simulink model "AirCtl_Gov"  (R2016b)
settings: configuration reference "CodeGenConfigSet" (kept outside this file)
values from neighbouring files (symbols this model uses):
  AirCtl_facParAirTemp_CUR = Calibration.Parameter    [init_AirCtl_Gov.m]    (also in init_AirCtl_Gov_SIL.m = Simulink.Parameter)
  AirCtl_facParAirTemp_CURX = Calibration.Parameter    [init_AirCtl_Gov.m]    (also in init_AirCtl_Gov_SIL.m = Simulink.Parameter)
  AirCtl_facParBas_MAP = Calibration.Parameter    [init_AirCtl_Gov.m]    (also in init_AirCtl_Gov_SIL.m = Simulink.Parameter)
  AirCtl_facParBas_MAPX = Calibration.Parameter    [init_AirCtl_Gov.m]    (also in init_AirCtl_Gov_SIL.m = Simulink.Parameter)
  AirCtl_facParBas_MAPY = Calibration.Parameter    [init_AirCtl_Gov.m]    (also in init_AirCtl_Gov_SIL.m = Simulink.Parameter)
  AirCtl_KdNrm_C = Calibration.Parameter    [init_AirCtl_Gov.m]    (also in init_AirCtl_Gov_SIL.m = Simulink.Parameter)
  AirCtl_KIconv_C = Calibration.Parameter    [init_AirCtl_Gov.m]    (also in init_AirCtl_Gov_SIL.m = Simulink.Parameter)
  AirCtl_KiNegNrm_C = Calibration.Parameter    [init_AirCtl_Gov.m]    (also in init_AirCtl_Gov_SIL.m = Simulink.Parameter)
  AirCtl_KiNrm_C = Calibration.Parameter    [init_AirCtl_Gov.m]    (also in init_AirCtl_Gov_SIL.m = Simulink.Parameter)
  AirCtl_KiPosNrm_C = Calibration.Parameter    [init_AirCtl_Gov.m]    (also in init_AirCtl_Gov_SIL.m = Simulink.Parameter)
  AirCtl_KiWinNegNrm_C = Calibration.Parameter    [init_AirCtl_Gov.m]    (also in init_AirCtl_Gov_SIL.m = Simulink.Parameter)
  AirCtl_KiWinPosNrm_C = Calibration.Parameter    [init_AirCtl_Gov.m]    (also in init_AirCtl_Gov_SIL.m = Simulink.Parameter)
  AirCtl_KpNegNrm_C = Calibration.Parameter    [init_AirCtl_Gov.m]    (also in init_AirCtl_Gov_SIL.m = Simulink.Parameter)
  AirCtl_KpNrm_C = Calibration.Parameter    [init_AirCtl_Gov.m]    (also in init_AirCtl_Gov_SIL.m = Simulink.Parameter)
  AirCtl_KpPosNrm_C = Calibration.Parameter    [init_AirCtl_Gov.m]    (also in init_AirCtl_Gov_SIL.m = Simulink.Parameter)
  AirCtl_KpWinNegNrm_C = Calibration.Parameter    [init_AirCtl_Gov.m]    (also in init_AirCtl_Gov_SIL.m = Simulink.Parameter)
  AirCtl_KpWinPosNrm_C = Calibration.Parameter    [init_AirCtl_Gov.m]    (also in init_AirCtl_Gov_SIL.m = Simulink.Parameter)
  AirCtl_numAirTempGov_C = Calibration.Parameter    [init_AirCtl_Gov.m]    (also in init_AirCtl_Gov_SIL.m = Simulink.Parameter)
  AirCtl_rEGR_MAP = Calibration.Parameter    [init_AirCtl_Gov.m]    (also in init_AirCtl_Gov_SIL.m = Simulink.Parameter)
  AirCtl_rEGR_MAPX = Calibration.Parameter    [init_AirCtl_Gov.m]    (also in init_AirCtl_Gov_SIL.m = Simulink.Parameter)
  AirCtl_rEGR_MAPY = Calibration.Parameter    [init_AirCtl_Gov.m]    (also in init_AirCtl_Gov_SIL.m = Simulink.Parameter)
  AirCtl_rGovMax_C = Calibration.Parameter    [init_AirCtl_Gov.m]    (also in init_AirCtl_Gov_SIL.m = Simulink.Parameter)
  AirCtl_rGovMin_C = Calibration.Parameter    [init_AirCtl_Gov.m]    (also in init_AirCtl_Gov_SIL.m = Simulink.Parameter)
  AirCtl_rIGovLimHi_C = Calibration.Parameter    [init_AirCtl_Gov.m]    (also in init_AirCtl_Gov_SIL.m = Simulink.Parameter)
  AirCtl_rIGovLimLo_C = Calibration.Parameter    [init_AirCtl_Gov.m]    (also in init_AirCtl_Gov_SIL.m = Simulink.Parameter)
  AirCtl_rTransCor_MAP = Calibration.Parameter    [init_AirCtl_Gov.m]    (also in init_AirCtl_Gov_SIL.m = Simulink.Parameter)
  AirCtl_rTransCor_MAPX = Calibration.Parameter    [init_AirCtl_Gov.m]    (also in init_AirCtl_Gov_SIL.m = Simulink.Parameter)
  AirCtl_rTransCor_MAPY = Calibration.Parameter    [init_AirCtl_Gov.m]    (also in init_AirCtl_Gov_SIL.m = Simulink.Parameter)
  AirCtl_rTVA_MAP = Calibration.Parameter    [init_AirCtl_Gov.m]    (also in init_AirCtl_Gov_SIL.m = Simulink.Parameter)
  AirCtl_rTVA_MAPX = Calibration.Parameter    [init_AirCtl_Gov.m]    (also in init_AirCtl_Gov_SIL.m = Simulink.Parameter)
  AirCtl_rTVA_MAPY = Calibration.Parameter    [init_AirCtl_Gov.m]    (also in init_AirCtl_Gov_SIL.m = Simulink.Parameter)
  AirCtl_stGov_C = Calibration.Parameter    [init_AirCtl_Gov.m]    (also in init_AirCtl_Gov_SIL.m = Simulink.Parameter)
  AirCtl_T1Nrm_C = Calibration.Parameter    [init_AirCtl_Gov.m]    (also in init_AirCtl_Gov_SIL.m = Simulink.Parameter)
undefined symbols (not defined in the file or in its folder): AirCtl_Gov_DT
libraries: CXLib x4
settings Model: Creator=Wollf  LastModifiedBy=zhulinfeng
settings ConfigSetRef: SourceLocation=Base Workspace

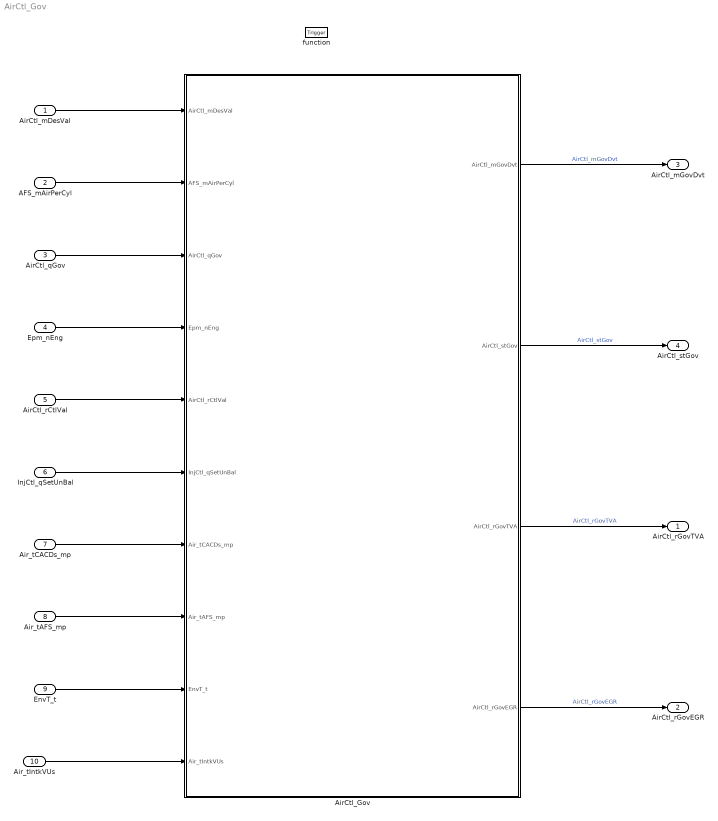
== system AirCtl_Gov ==
  AirCtl_mDesVal : Inport  Tag=mg/hub  Description=Desired air mass  OutMin=-15000  OutMax=15000  OutDataTypeStr=AirMass_mg_hub
  AFS_mAirPerCyl : Inport  Tag=mg/hub  Description=Air mass per cylinder  Port=2  OutMin=0  OutMax=16383  OutDataTypeStr=AirMass_mg_hub
  AirCtl_qGov : Inport  Tag=mg/hub  Description=Inner quantity for open-loop control of the exhaustgas recirculation control  Port=3  OutMin=-319  OutMax=319  OutDataTypeStr=FuelMass_mg_hub
  Epm_nEng : Inport  Tag=rpm  Description=Engine speed  Port=4  OutMin=0  OutMax=6000  OutDataTypeStr=EngSpeed_rpm
  AirCtl_rCtlVal : Inport  Tag=%  Description=Stationary part of controlled variable  Port=5  OutMin=-100  OutMax=100  OutDataTypeStr=Prc_100_rate
  InjCtl_qSetUnBal : Inport  Tag=mg/hub  Description=Current injection quantity  Port=6  OutMin=-319  OutMax=319  OutDataTypeStr=FuelMass_mg_hub
  Air_tCACDs_mp : Inport  Tag=deg  Description=Charge-air temperature downstream from charge-air cooler  Port=7  OutMin=-200  OutMax=200  OutDataTypeStr=Temp_deg
  Air_tAFS_mp : Inport  Tag=deg  Description=Induction air temperature at the HFM  Port=8  OutMin=-200  OutMax=200  OutDataTypeStr=Temp_deg
  EnvT_t : Inport  Tag=deg  Description=Environmental temperature  Port=9  OutMin=-200  OutMax=200  OutDataTypeStr=Temp_deg
  Air_tIntkVUs : Inport  Tag=deg  Description=Intake air temperature upstream of the inlet valve  Port=10  OutMin=-200  OutMax=200  OutDataTypeStr=Temp_deg
  function : TriggerPort  TriggerType=function-call  VariantControl=Variant
  AirCtl_Gov : Subsystem
  AirCtl_rGovTVA : Outport  Tag=%  Description=Opening for intake throttle (TVA)  OutMin=-100  OutMax=100  OutDataTypeStr=Prc_100_rate
  AirCtl_rGovEGR : Outport  Tag=%  Description=Setpoint position of the exhaust-gas recirculation valve from the exhaust-gas recirculation control  Port=2  OutMin=-100  OutMax=100  OutDataTypeStr=Prc_100_rate
  AirCtl_mGovDvt : Outport  Tag=mg/hub  Description=Deviation of Air mass  Port=3  OutMin=-15000  OutMax=15000  OutDataTypeStr=AirMass_mg_hub
  AirCtl_stGov : Outport  Description=Status of the exhaust-gas recirculation control  Port=4  OutMin=0  OutMax=255  OutDataTypeStr=State_uint8
  wires:
  AirCtl_mDesVal/1 -> AirCtl_Gov/1(AirCtl_mDesVal)
  AFS_mAirPerCyl/1 -> AirCtl_Gov/2(AFS_mAirPerCyl)
  AirCtl_qGov/1 -> AirCtl_Gov/3(AirCtl_qGov)
  Epm_nEng/1 -> AirCtl_Gov/4(Epm_nEng)
  AirCtl_rCtlVal/1 -> AirCtl_Gov/5(AirCtl_rCtlVal)
  InjCtl_qSetUnBal/1 -> AirCtl_Gov/6(InjCtl_qSetUnBal)
  Air_tCACDs_mp/1 -> AirCtl_Gov/7(Air_tCACDs_mp)
  Air_tAFS_mp/1 -> AirCtl_Gov/8(Air_tAFS_mp)
  EnvT_t/1 -> AirCtl_Gov/9(EnvT_t)
  Air_tIntkVUs/1 -> AirCtl_Gov/10(Air_tIntkVUs)
  AirCtl_Gov/1(AirCtl_mGovDvt) -> AirCtl_mGovDvt/1  "AirCtl_mGovDvt"
  AirCtl_Gov/2(AirCtl_stGov) -> AirCtl_stGov/1  "AirCtl_stGov"
  AirCtl_Gov/3(AirCtl_rGovTVA) -> AirCtl_rGovTVA/1  "AirCtl_rGovTVA"
  AirCtl_Gov/4(AirCtl_rGovEGR) -> AirCtl_rGovEGR/1  "AirCtl_rGovEGR"

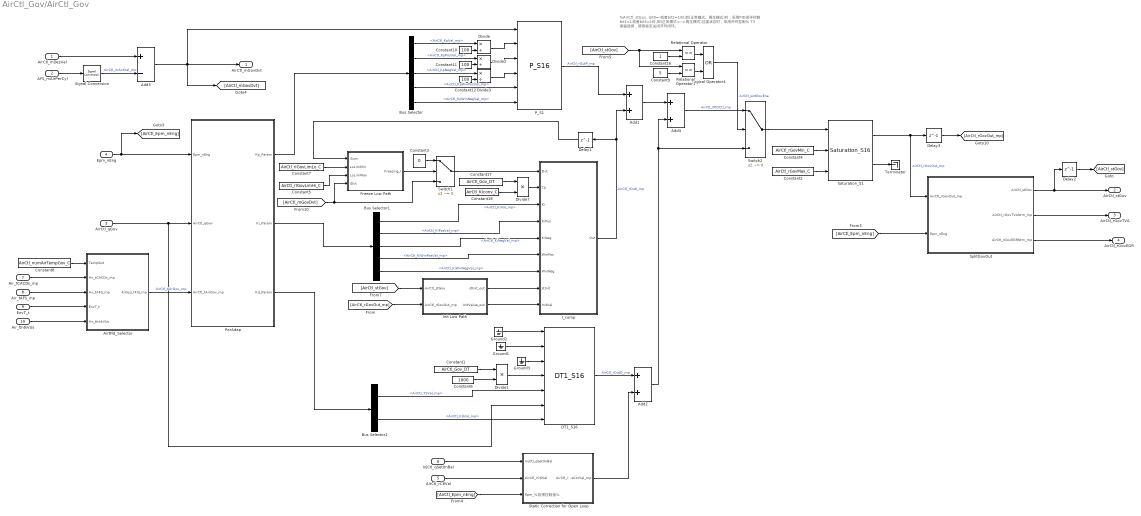
== system AirCtl_Gov/AirCtl_Gov ==
  note: %AirCtl_stGov,
      | bit0=1或者bit2=1时,即(正常模式、再生模式)时，采用PID闭环控制
      | bit1=1或者bit3=1时,即(正常模式<-->再生模式)过渡状态时，采用开环控制%
      | T3 保留选择，使用标定关闭开环闭环。
  note: %前馈控制值%
  AirCtl_mDesVal : Inport  Tag=mg/hub  Description=Desired air mass  OutDataTypeStr=AirMass_mg_hub
  AFS_mAirPerCyl : Inport  Tag=mg/hub  Description=Air mass per cylinder  Port=2
  AirCtl_qGov : Inport  Tag=mg/hub  Description=Inner quantity for open-loop control of the exhaustgas recirculation control  Port=3
  Epm_nEng : Inport  Tag=rpm  Description=Engine speed  Port=4
  AirCtl_rCtlVal : Inport  Tag=%  Description=Stationary part of controlled variable  Port=5
  InjCtl_qSetUnBal : Inport  Tag=mg/hub  Description=Current injection quantity  Port=6
  Air_tCACDs_mp : Inport  Tag=deg  Description=Charge-air temperature downstream from charge-air cooler  Port=7
  Air_tAFS_mp : Inport  Tag=deg  Description=Induction air temperature at the HFM  Port=8
  EnvT_t : Inport  Tag=deg  Description=Environmental temperature  Port=9
  Air_tIntkVUs : Inport  Tag=deg  Description=Intake air temperature upstream of the inlet valve  Port=10
  Add1 : Sum  SaturateOnIntegerOverflow=on  InputSameDT=on
  Add2 : Sum  SaturateOnIntegerOverflow=on  InputSameDT=on
  Add3 : Sum  Inputs=+-  SaturateOnIntegerOverflow=on  InputSameDT=on
  Add4 : Sum  SaturateOnIntegerOverflow=on  InputSameDT=on
  AirtFld_Selector : Subsystem
  Bus Selector : BusSelector  OutputSignals=AirCtl_KpVal_mp,AirCtl_KpPosVal_mp,AirCtl_KpNegVal_mp,AirCtl_KpWinPosVal_mp,AirCtl_KpWinNegVal_mp
  Bus Selector1 : BusSelector  OutputSignals=AirCtl_KiVal_mp,AirCtl_KiPosVal_mp,AirCtl_KiNegVal_mp,AirCtl_KiWinPosVal_mp,AirCtl_KiWinNegVal_mp
  Bus Selector2 : BusSelector  OutputSignals=AirCtl_T1Val_mp,AirCtl_KdVal_mp
  Constant1 : Constant  Value=AirCtl_Gov_DT
  Constant10 : Constant  Value=100  OutDataTypeStr=uint8
  Constant11 : Constant  Value=100  OutDataTypeStr=uint8
  Constant12 : Constant  Value=100  OutDataTypeStr=uint8
  Constant16 : Constant  OutDataTypeStr=Inherit: Inherit via back propagation
  Constant17 : Constant  Value=AirCtl_Gov_DT
  Constant18 : Constant  Value=AirCtl_KIconv_C
  Constant2 : Constant  Value=AirCtl_rGovMax_C
  Constant3 : Constant  Value=0  OutDataTypeStr=Inherit: Inherit via back propagation
  Constant4 : Constant  Value=AirCtl_rGovMin_C
  Constant5 : Constant  Value=AirCtl_rIGovLimHi_C
  Constant6 : Constant  Value=1000  OutDataTypeStr=uint32
  Constant7 : Constant  Value=AirCtl_rIGovLimLo_C
  Constant8 : Constant  Value=AirCtl_numAirTempGov_C
  Constant9 : Constant  Value=5  OutDataTypeStr=Inherit: Inherit via back propagation
  DT1_S16 : CXLib/DT1_S16
  Delay1 : Delay  DelayLength=1  InitialCondition=0
  Delay2 : Delay  DelayLength=1  InitialCondition=0
  Delay3 : Delay  DelayLength=1  InitialCondition=0
  Divide : Product  Inputs=*/  OutDataTypeStr=fixdt(1,32,2^-14,0)  SaturateOnIntegerOverflow=on
  Divide1 : Product  Inputs=**  OutDataTypeStr=Inherit: Inherit via back propagation  SaturateOnIntegerOverflow=on
  Divide2 : Product  Inputs=*/  OutDataTypeStr=fixdt(1,32,2^-14,0)  SaturateOnIntegerOverflow=on
  Divide3 : Product  Inputs=*/  OutDataTypeStr=fixdt(1,32,2^-14,0)  SaturateOnIntegerOverflow=on
  Divide7 : Product  Inputs=**  SaturateOnIntegerOverflow=on  OutDataTypeStr=Inherit: Same as first input
  Freeze Low Path : Subsystem
  Ground1 : Ground
  Ground2 : Ground
  Ground3 : Ground
  I_comp : Subsystem
  Init Low Path : Subsystem
  Logical Operator4 : Logic  Operator=OR  OutDataTypeStr=boolean
  P_S1 : CXLib/P_S16
  ParAdap : Subsystem
  Relational Operator : RelationalOperator  Operator===  OutDataTypeStr=boolean  RndMeth=Simplest
  Relational Operator1 : RelationalOperator  Operator===  OutDataTypeStr=boolean  RndMeth=Simplest
  Saturation_S1 : CXLib/Saturation_S16
  Signal Conversion : SignalConversion  OverrideOpt=off
  SplitGovOut : Subsystem
  Static Correction for Open Loop : Subsystem
  Switch1 : Switch  Criteria=u2 ~= 0  SaturateOnIntegerOverflow=on  InputSameDT=on
  Switch2 : Switch  Criteria=u2 ~= 0  SaturateOnIntegerOverflow=on  InputSameDT=on
  Terminator : Terminator
  AirCtl_mGovDvt : Outport  Tag=mg/hub  Description=Deviation of Air mass
  AirCtl_stGov : Outport  Description=Status of the exhaust-gas recirculation control  Port=2
  AirCtl_rGovTVA : Outport  Tag=%  Description=Opening for intake throttle (TVA)  Port=3
  AirCtl_rGovEGR : Outport  Tag=%  Description=Setpoint position of the exhaust-gas recirculation valve from the exhaust-gas recirculation control  Port=4
  wires:
  I_comp/1(Out) -> Add1/2, Delay1/1  "AirCtl_rOutI_mp"
  Bus Selector/1 -> Divide/1  "<AirCtl_KpVal_mp>"
  Static Correction for Open Loop/1(AirCtl_rTransCorVal_mp) -> Add2/2
  Bus Selector2/2 -> DT1_S16/7  "<AirCtl_KdVal_mp>"
  ParAdap/2(Ki_Param) -> Bus Selector1/1
  AirCtl_mDesVal/1 -> Add3/1
  ParAdap/1(Kp_Param) -> Bus Selector/1
  Delay1/1 -> Freeze Low Path/1(iSum)
  Constant6/1 -> Divide1/2
  Constant1/1 -> Divide1/1
  Delay3/1 -> [AirCtl_rGovOut_mp]
  Logical Operator4/1 -> Switch2/2  "AirCtl_swtGovEna"
  Constant5/1 -> Freeze Low Path/3(LoLimMax)
  [AirCtl_rGovOut_mp] -> Init Low Path/2(AirCtl_rGovOut_mp)
  [AirCtl_stGov] -> Init Low Path/1(AirCtl_stGov)
  [AirCtl_stGov] -> Relational Operator1/1, Relational Operator/1
  Constant7/1 -> Freeze Low Path/2(LoLimMin)
  Init Low Path/1(stInit_out) -> I_comp/8(stInit)
  Switch1/1 -> I_comp/1(Dvt)
  Init Low Path/2(InitValue_out) -> I_comp/9(InitVal)
  [AirCtl_Epm_nEng] -> Static Correction for Open Loop/3(Epm_nEng)
  Constant2/1 -> Saturation_S1/3
  Divide1/1 -> DT1_S16/4
  InjCtl_qSetUnBal/1 -> Static Correction for Open Loop/1(InjCtl_qSetUnBal)
  AFS_mAirPerCyl/1 -> Signal Conversion/1
  Add3/1 -> P_S1/1, [AirCtl_mGovDvt], AirCtl_mGovDvt/1
  Add4/1 -> Switch2/1  "AirCtl_rPIDCtl_mp"
  Constant3/1 -> Switch1/1
  Ground1/1 -> DT1_S16/2
  [AirCtl_mGovDvt] -> Switch1/3, Freeze Low Path/4(iDvt)
  Saturation_S1/2 -> Terminator/1
  Freeze Low Path/1(Freezing_I) -> Switch1/2
  Add2/1 -> Add4/2, Switch2/3
  Bus Selector2/1 -> DT1_S16/5  "<AirCtl_T1Val_mp>"
  Add1/1 -> Add4/1
  Bus Selector/3 -> Divide3/1  "<AirCtl_KpNegVal_mp>"
  Bus Selector/5 -> P_S1/6  "<AirCtl_KpWinNegVal_mp>"
  Bus Selector/4 -> P_S1/5  "<AirCtl_KpWinPosVal_mp>"
  Constant4/1 -> Saturation_S1/2
  Switch2/1 -> Saturation_S1/1
  AirCtl_rCtlVal/1 -> Static Correction for Open Loop/2(AirCtl_rCtlVal)
  [AirCtl_Epm_nEng] -> SplitGovOut/2(Epm_nEng)
  Saturation_S1/1 -> SplitGovOut/1(AirCtl_rGovOut_mp), Delay3/1  "AirCtl_rGovOut_mp"
  Bus Selector1/5 -> I_comp/7(WinNeg)  "<AirCtl_KiWinNegVal_mp>"
  Bus Selector1/1 -> I_comp/3(Ki)  "<AirCtl_KiVal_mp>"
  Bus Selector1/2 -> I_comp/4(KiPos)  "<AirCtl_KiPosVal_mp>"
  DT1_S16/1 -> Add2/1  "AirCtl_rOutD_mp"
  AirtFld_Selector/1(AirSys_tFld_mp) -> ParAdap/3(AirCtl_tAirGov_mp)  "AirCtl_tAirGov_mp"
  Air_tAFS_mp/1 -> AirtFld_Selector/3(Air_tAFS_mp)
  Air_tIntkVUs/1 -> AirtFld_Selector/5(Air_tIntkVUs)
  P_S1/1 -> Add1/1  "AirCtl_rOutP_mp"
  Bus Selector1/3 -> I_comp/5(KiNeg)  "<AirCtl_KiNegVal_mp>"
  ParAdap/3(Kd_Param) -> Bus Selector2/1
  Signal Conversion/1 -> Add3/2  "AirCtl_mActVal_mp"
  Ground2/1 -> DT1_S16/1
  Ground3/1 -> DT1_S16/3
  Bus Selector/2 -> Divide2/1  "<AirCtl_KpPosVal_mp>"
  Constant8/1 -> AirtFld_Selector/1(TempSwt)
  Air_tCACDs_mp/1 -> AirtFld_Selector/2(Air_tCACDs_mp)
  Bus Selector1/4 -> I_comp/6(WinPos)  "<AirCtl_KiWinPosVal_mp>"
  AirCtl_qGov/1 -> DT1_S16/6, ParAdap/2(AirCtl_qGov)
  EnvT_t/1 -> AirtFld_Selector/4(EnvT_t)
  Epm_nEng/1 -> [AirCtl_Epm_nEng], ParAdap/1(Epm_nEng)
  SplitGovOut/1(AirCtl_stGov) -> Delay2/1, AirCtl_stGov/1
  Divide/1 -> P_S1/2
  Constant10/1 -> Divide/2
  SplitGovOut/2(AirCtl_rGovTVANrm_mp) -> AirCtl_rGovTVA/1
  Divide3/1 -> P_S1/4
  Divide2/1 -> P_S1/3
  Delay2/1 -> [AirCtl_stGov]
  SplitGovOut/3(AirCtl_rGovEGRNrm_mp) -> AirCtl_rGovEGR/1
  Constant11/1 -> Divide2/2
  Constant12/1 -> Divide3/2
  Constant16/1 -> Relational Operator/2
  Relational Operator/1 -> Logical Operator4/1
  Constant9/1 -> Relational Operator1/2
  Relational Operator1/1 -> Logical Operator4/2
  Constant18/1 -> Divide7/2
  Constant17/1 -> Divide7/1
  Divide7/1 -> I_comp/2(T0)

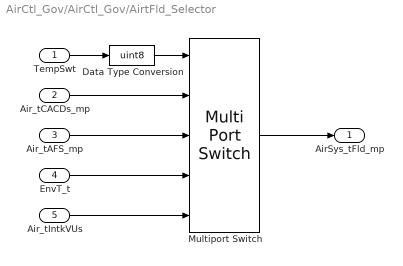
== system AirCtl_Gov/AirCtl_Gov/AirtFld_Selector ==
  TempSwt : Inport
  Air_tCACDs_mp : Inport  Tag=deg  Description=Charge-air temperature downstream from charge-air cooler  Port=2
  Air_tAFS_mp : Inport  Tag=deg  Description=Induction air temperature at the HFM  Port=3
  EnvT_t : Inport  Tag=deg  Description=Environmental temperature  Port=4
  Air_tIntkVUs : Inport  Tag=deg  Description=Intake air temperature upstream of the inlet valve  Port=5
  Data Type Conversion : DataTypeConversion  OutDataTypeStr=uint8
  Multiport Switch : MultiPortSwitch  DataPortOrder=Zero-based contiguous  Inputs=4
  AirSys_tFld_mp : Outport  Tag=deg  Description=Engine temperature field
  wires:
  Air_tCACDs_mp/1 -> Multiport Switch/2
  Multiport Switch/1 -> AirSys_tFld_mp/1
  EnvT_t/1 -> Multiport Switch/4
  Air_tAFS_mp/1 -> Multiport Switch/3
  Data Type Conversion/1 -> Multiport Switch/1
  TempSwt/1 -> Data Type Conversion/1
  Air_tIntkVUs/1 -> Multiport Switch/5

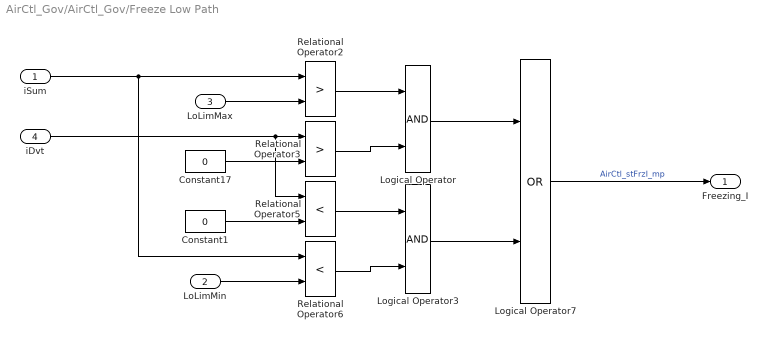
== system AirCtl_Gov/AirCtl_Gov/Freeze Low Path ==
  iSum : Inport
  LoLimMin : Inport  Port=2
  LoLimMax : Inport  Port=3
  iDvt : Inport  Port=4
  Constant1 : Constant  Value=0  OutDataTypeStr=Inherit: Inherit via back propagation  SampleTime=-1
  Constant17 : Constant  Value=0  OutDataTypeStr=Inherit: Inherit via back propagation  SampleTime=-1
  Logical Operator : Logic  AllPortsSameDT=off  OutDataTypeStr=boolean
  Logical Operator3 : Logic  AllPortsSameDT=off  OutDataTypeStr=boolean
  Logical Operator7 : Logic  Operator=OR  OutDataTypeStr=boolean
  Relational Operator2 : RelationalOperator  Operator=>  OutDataTypeStr=boolean  RndMeth=Nearest  InputSameDT=on
  Relational Operator3 : RelationalOperator  Operator=>  OutDataTypeStr=boolean  RndMeth=Nearest  InputSameDT=on
  Relational Operator5 : RelationalOperator  Operator=<  OutDataTypeStr=boolean  RndMeth=Nearest  InputSameDT=on
  Relational Operator6 : RelationalOperator  Operator=<  OutDataTypeStr=boolean  RndMeth=Nearest  InputSameDT=on
  Freezing_I : Outport
  wires:
  iSum/1 -> Relational Operator2/1, Relational Operator6/1
  Logical Operator3/1 -> Logical Operator7/2
  Logical Operator/1 -> Logical Operator7/1
  Constant1/1 -> Relational Operator5/2
  LoLimMax/1 -> Relational Operator2/2
  iDvt/1 -> Relational Operator3/1, Relational Operator5/1
  Constant17/1 -> Relational Operator3/2
  LoLimMin/1 -> Relational Operator6/2
  Relational Operator2/1 -> Logical Operator/1
  Relational Operator3/1 -> Logical Operator/2
  Relational Operator5/1 -> Logical Operator3/1
  Logical Operator7/1 -> Freezing_I/1  "AirCtl_stFrzI_mp"
  Relational Operator6/1 -> Logical Operator3/2

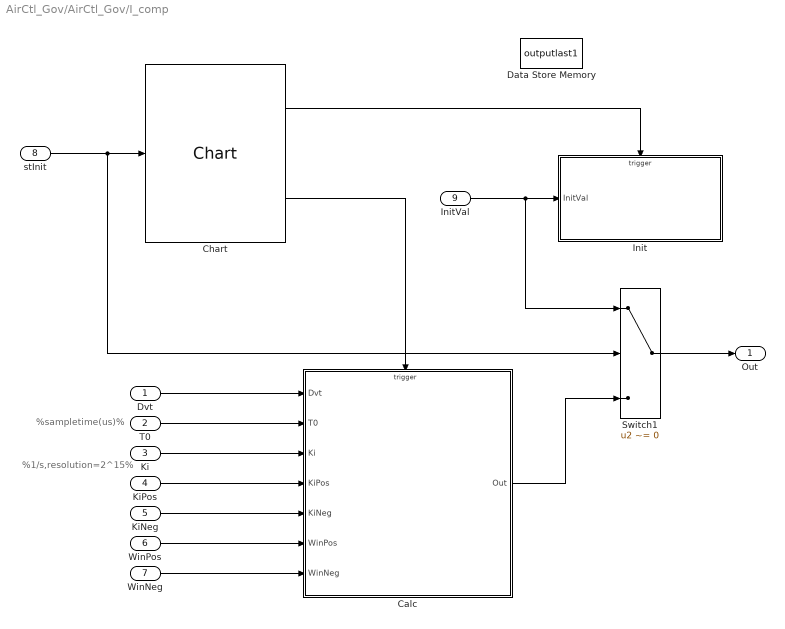
== system AirCtl_Gov/AirCtl_Gov/I_comp ==
  note: %sampletime(us)%
  note: %1/s,resolution=2^15%
  Dvt : Inport
  T0 : Inport  Port=2  OutDataTypeStr=uint32
  Ki : Inport  Port=3
  KiPos : Inport  Port=4
  KiNeg : Inport  Port=5
  WinPos : Inport  Port=6
  WinNeg : Inport  Port=7
  stInit : Inport  Port=8  OutDataTypeStr=boolean
  InitVal : Inport  Port=9
  Calc : Subsystem
  Chart : CXLib/I_S16/Chart
  Data Store Memory : DataStoreMemory  DataStoreName=outputlast1  ReadBeforeWriteMsg=warning  WriteAfterWriteMsg=warning  WriteAfterReadMsg=warning  ShowAdditionalParam=off  OutDataTypeStr=fixdt(1,16,2^-7,0)
  Init : Subsystem
  Switch1 : Switch  Criteria=u2 ~= 0  SaturateOnIntegerOverflow=on  InputSameDT=on
  Out : Outport
  wires:
  Chart/1 -> Init/Trigger
  stInit/1 -> Chart/1, Switch1/2
  Ki/1 -> Calc/3(Ki)
  Dvt/1 -> Calc/1(Dvt)
  T0/1 -> Calc/2(T0)
  Calc/1(Out) -> Switch1/3
  KiNeg/1 -> Calc/5(KiNeg)
  Switch1/1 -> Out/1
  Chart/2 -> Calc/Trigger
  WinNeg/1 -> Calc/7(WinNeg)
  InitVal/1 -> Init/1(InitVal), Switch1/1
  WinPos/1 -> Calc/6(WinPos)
  KiPos/1 -> Calc/4(KiPos)

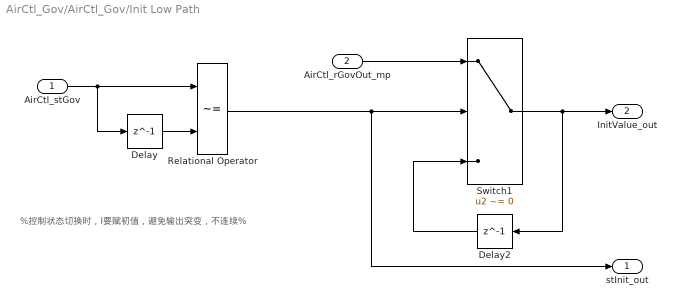
== system AirCtl_Gov/AirCtl_Gov/Init Low Path ==
  note: %控制状态切换时，I要赋初值，避免输出突变，不连续%
  AirCtl_stGov : Inport
  AirCtl_rGovOut_mp : Inport  Port=2
  Delay : Delay  DelayLength=1  InitialCondition=0
  Delay2 : Delay  DelayLength=1  InitialCondition=0
  Relational Operator : RelationalOperator  Operator=~=  OutDataTypeStr=boolean  RndMeth=Simplest  InputSameDT=on
  Switch1 : Switch  Criteria=u2 ~= 0  SaturateOnIntegerOverflow=on  InputSameDT=on
  stInit_out : Outport
  InitValue_out : Outport  Port=2
  wires:
  Delay/1 -> Relational Operator/2
  AirCtl_stGov/1 -> Relational Operator/1, Delay/1
  AirCtl_rGovOut_mp/1 -> Switch1/1
  Delay2/1 -> Switch1/3
  Relational Operator/1 -> stInit_out/1, Switch1/2
  Switch1/1 -> Delay2/1, InitValue_out/1

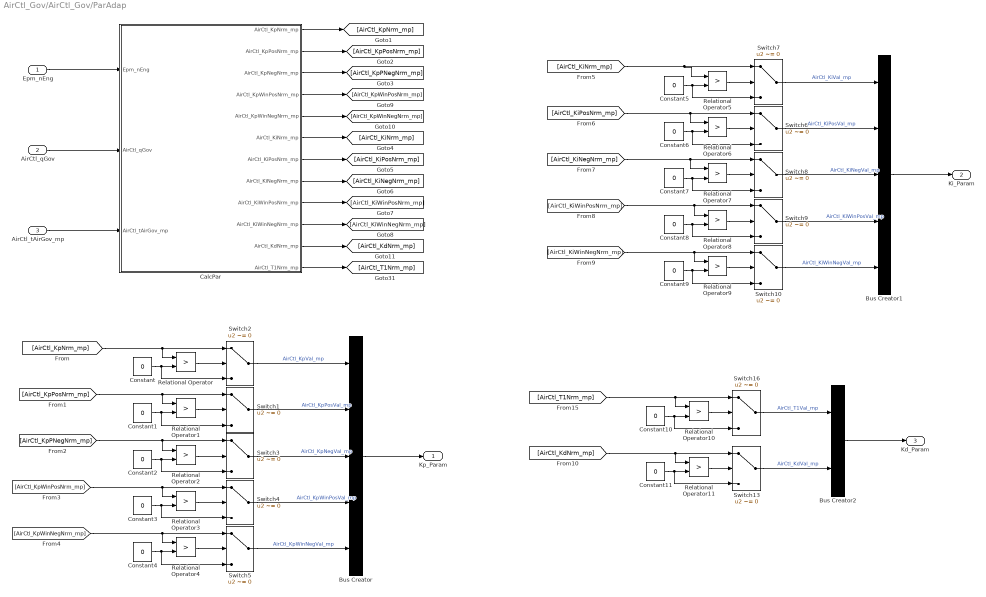
== system AirCtl_Gov/AirCtl_Gov/ParAdap ==
  Epm_nEng : Inport
  AirCtl_qGov : Inport  Port=2
  AirCtl_tAirGov_mp : Inport  Port=3
  Bus Creator : BusCreator  Inputs=5
  Bus Creator1 : BusCreator  Inputs=5
  Bus Creator2 : BusCreator  Inputs=2
  CalcPar : Subsystem
  Constant{,1..11} (12 alike) : Constant  Value=0  OutDataTypeStr=Inherit: Inherit via back propagation
  Relational Operator{,1..11} (12 alike) : RelationalOperator  Operator=>  OutDataTypeStr=boolean  RndMeth=Simplest
  Switch{1..10,13,16} (12 alike) : Switch  Criteria=u2 ~= 0  SaturateOnIntegerOverflow=on  InputSameDT=on
  Kp_Param : Outport
  Ki_Param : Outport  Port=2
  Kd_Param : Outport  Port=3
  wires:
  CalcPar/12(AirCtl_T1Nrm_mp) -> [AirCtl_T1Nrm_mp]
  CalcPar/11(AirCtl_KdNrm_mp) -> [AirCtl_KdNrm_mp]
  CalcPar/10(AirCtl_KiWinNegNrm_mp) -> [AirCtl_KiWinNegNrm_mp]
  CalcPar/9(AirCtl_KiWinPosNrm_mp) -> [AirCtl_KiWinPosNrm_mp]
  CalcPar/8(AirCtl_KiNegNrm_mp) -> [AirCtl_KiNegNrm_mp]
  CalcPar/7(AirCtl_KiPosNrm_mp) -> [AirCtl_KiPosNrm_mp]
  CalcPar/6(AirCtl_KiNrm_mp) -> [AirCtl_KiNrm_mp]
  CalcPar/5(AirCtl_KpWinNegNrm_mp) -> [AirCtl_KpWinNegNrm_mp]
  CalcPar/4(AirCtl_KpWinPosNrm_mp) -> [AirCtl_KpWinPosNrm_mp]
  CalcPar/3(AirCtl_KpNegNrm_mp) -> [AirCtl_KpPNegNrm_mp]
  CalcPar/2(AirCtl_KpPosNrm_mp) -> [AirCtl_KpPosNrm_mp]
  CalcPar/1(AirCtl_KpNrm_mp) -> [AirCtl_KpNrm_mp]
  Switch16/1 -> Bus Creator2/1  "AirCtl_T1Val_mp"
  Bus Creator2/1 -> Kd_Param/1
  Bus Creator1/1 -> Ki_Param/1
  Switch13/1 -> Bus Creator2/2  "AirCtl_KdVal_mp"
  Switch10/1 -> Bus Creator1/5  "AirCtl_KiWinNegVal_mp"
  Switch9/1 -> Bus Creator1/4  "AirCtl_KiWinPosVal_mp"
  Switch8/1 -> Bus Creator1/3  "AirCtl_KiNegVal_mp"
  Switch6/1 -> Bus Creator1/2  "AirCtl_KiPosVal_mp"
  Switch7/1 -> Bus Creator1/1  "AirCtl_KiVal_mp"
  Switch5/1 -> Bus Creator/5  "AirCtl_KpWinNegVal_mp"
  Switch4/1 -> Bus Creator/4  "AirCtl_KpWinPosVal_mp"
  Switch3/1 -> Bus Creator/3  "AirCtl_KpNegVal_mp"
  Switch1/1 -> Bus Creator/2  "AirCtl_KpPosVal_mp"
  Switch2/1 -> Bus Creator/1  "AirCtl_KpVal_mp"
  Bus Creator/1 -> Kp_Param/1
  [AirCtl_KpNrm_mp] -> Relational Operator/1, Switch2/1
  AirCtl_qGov/1 -> CalcPar/2(AirCtl_qGov)
  AirCtl_tAirGov_mp/1 -> CalcPar/3(AirCtl_tAirGov_mp)
  Epm_nEng/1 -> CalcPar/1(Epm_nEng)
  Relational Operator/1 -> Switch2/2
  Constant/1 -> Switch2/3, Relational Operator/2
  [AirCtl_KpPosNrm_mp] -> Switch1/1, Relational Operator1/1
  Relational Operator1/1 -> Switch1/2
  Constant1/1 -> Switch1/3, Relational Operator1/2
  [AirCtl_KpPNegNrm_mp] -> Switch3/1, Relational Operator2/1
  Relational Operator2/1 -> Switch3/2
  Constant2/1 -> Switch3/3, Relational Operator2/2
  [AirCtl_KpWinPosNrm_mp] -> Switch4/1, Relational Operator3/1
  Relational Operator3/1 -> Switch4/2
  Constant3/1 -> Switch4/3, Relational Operator3/2
  [AirCtl_KpWinNegNrm_mp] -> Switch5/1, Relational Operator4/1
  Relational Operator4/1 -> Switch5/2
  Constant4/1 -> Switch5/3, Relational Operator4/2
  [AirCtl_KiNrm_mp] -> Switch7/1, Relational Operator5/1
  Relational Operator5/1 -> Switch7/2
  Constant5/1 -> Switch7/3, Relational Operator5/2
  [AirCtl_KiPosNrm_mp] -> Switch6/1, Relational Operator6/1
  Relational Operator6/1 -> Switch6/2
  Constant6/1 -> Switch6/3, Relational Operator6/2
  [AirCtl_KiNegNrm_mp] -> Switch8/1, Relational Operator7/1
  Relational Operator7/1 -> Switch8/2
  Constant7/1 -> Switch8/3, Relational Operator7/2
  [AirCtl_KiWinPosNrm_mp] -> Switch9/1, Relational Operator8/1
  Relational Operator8/1 -> Switch9/2
  Constant8/1 -> Switch9/3, Relational Operator8/2
  [AirCtl_KiWinNegNrm_mp] -> Switch10/1, Relational Operator9/1
  Relational Operator9/1 -> Switch10/2
  Constant9/1 -> Switch10/3, Relational Operator9/2
  [AirCtl_T1Nrm_mp] -> Relational Operator10/1, Switch16/1
  Relational Operator10/1 -> Switch16/2
  Constant10/1 -> Switch16/3, Relational Operator10/2
  [AirCtl_KdNrm_mp] -> Switch13/1, Relational Operator11/1
  Relational Operator11/1 -> Switch13/2
  Constant11/1 -> Switch13/3, Relational Operator11/2

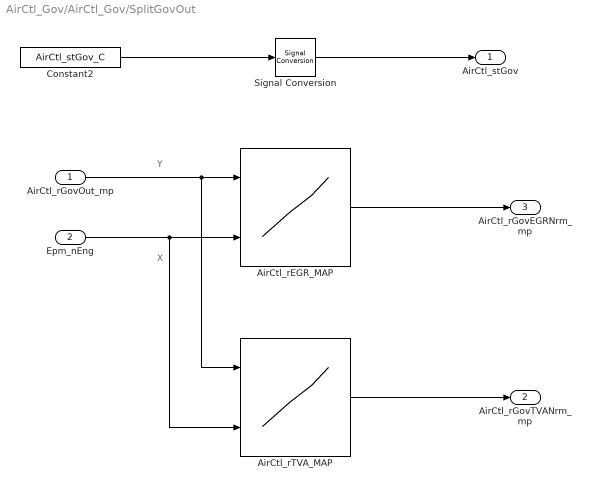
== system AirCtl_Gov/AirCtl_Gov/SplitGovOut ==
  note: Y
  note: X
  AirCtl_rGovOut_mp : Inport
  Epm_nEng : Inport  Port=2
  AirCtl_rEGR_MAP : Lookup_n-D  BreakpointsForDimension1=AirCtl_rEGR_MAPY  BreakpointsForDimension2=AirCtl_rEGR_MAPX  BeginIndexSearchUsingPreviousIndexResult=on  Table=AirCtl_rEGR_MAP  TableDataTypeStr=Inherit: Inherit from 'Table data'  ExtrapMethod=Clip  UseLastTableValue=on  InternalRulePriority=Speed  OutDataTypeStr=Inherit: Inherit from 'Table data'  RndMeth=Simplest  SaturateOnIntegerOverflow=on
  AirCtl_rTVA_MAP : Lookup_n-D  BreakpointsForDimension1=AirCtl_rTVA_MAPY  BreakpointsForDimension2=AirCtl_rTVA_MAPX  BeginIndexSearchUsingPreviousIndexResult=on  Table=AirCtl_rTVA_MAP  TableDataTypeStr=Inherit: Inherit from 'Table data'  ExtrapMethod=Clip  UseLastTableValue=on  InternalRulePriority=Speed  OutDataTypeStr=Inherit: Inherit from 'Table data'  RndMeth=Simplest  SaturateOnIntegerOverflow=on
  Constant2 : Constant  Value=AirCtl_stGov_C
  Signal Conversion : SignalConversion  OverrideOpt=off
  AirCtl_stGov : Outport
  AirCtl_rGovTVANrm_mp : Outport  Port=2
  AirCtl_rGovEGRNrm_mp : Outport  Port=3
  wires:
  AirCtl_rTVA_MAP/1 -> AirCtl_rGovTVANrm_mp/1
  AirCtl_rEGR_MAP/1 -> AirCtl_rGovEGRNrm_mp/1
  Epm_nEng/1 -> AirCtl_rEGR_MAP/2, AirCtl_rTVA_MAP/2
  AirCtl_rGovOut_mp/1 -> AirCtl_rEGR_MAP/1, AirCtl_rTVA_MAP/1
  Constant2/1 -> Signal Conversion/1
  Signal Conversion/1 -> AirCtl_stGov/1

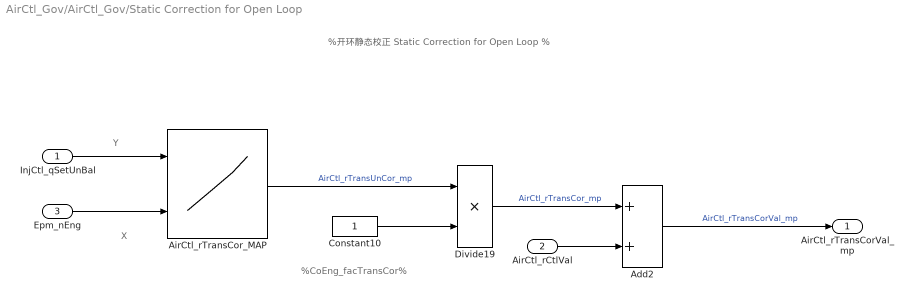
== system AirCtl_Gov/AirCtl_Gov/Static Correction for Open Loop ==
  note: %CoEng_facTransCor%
  note: %开环静态校正
      | Static Correction for Open Loop %
  note: X
  note: Y
  InjCtl_qSetUnBal : Inport
  AirCtl_rCtlVal : Inport  Port=2
  Epm_nEng : Inport  Port=3
  Add2 : Sum  SaturateOnIntegerOverflow=on  InputSameDT=on
  AirCtl_rTransCor_MAP : Lookup_n-D  BreakpointsForDimension1=AirCtl_rTransCor_MAPY  BreakpointsForDimension2=AirCtl_rTransCor_MAPX  BeginIndexSearchUsingPreviousIndexResult=on  Table=AirCtl_rTransCor_MAP  TableDataTypeStr=Inherit: Inherit from 'Table data'  ExtrapMethod=Clip  UseLastTableValue=on  InternalRulePriority=Speed  OutDataTypeStr=Inherit: Inherit from 'Table data'  RndMeth=Simplest  SaturateOnIntegerOverflow=on
  Constant10 : Constant  OutDataTypeStr=Factor
  Divide19 : Product  Inputs=**  OutDataTypeStr=Inherit: Inherit via back propagation  SaturateOnIntegerOverflow=on
  AirCtl_rTransCorVal_mp : Outport
  wires:
  Add2/1 -> AirCtl_rTransCorVal_mp/1  "AirCtl_rTransCorVal_mp"
  AirCtl_rCtlVal/1 -> Add2/2
  Divide19/1 -> Add2/1  "AirCtl_rTransCor_mp"
  Constant10/1 -> Divide19/2
  AirCtl_rTransCor_MAP/1 -> Divide19/1  "AirCtl_rTransUnCor_mp"
  Epm_nEng/1 -> AirCtl_rTransCor_MAP/2
  InjCtl_qSetUnBal/1 -> AirCtl_rTransCor_MAP/1

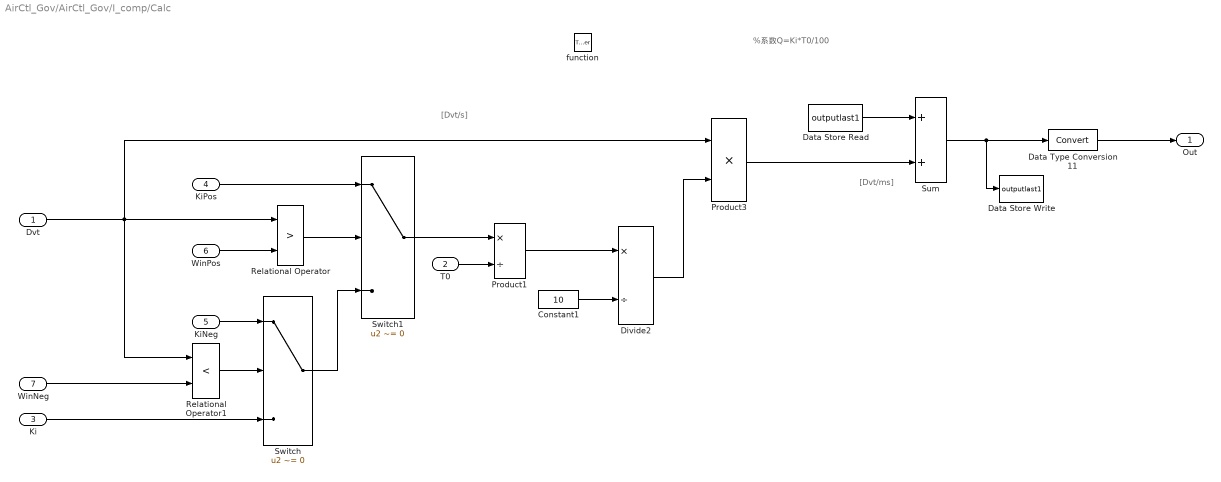
== system AirCtl_Gov/AirCtl_Gov/I_comp/Calc ==
  note: %系数Q=Ki*T0/100
  note: [Dvt/s]
  note: [Dvt/ms]
  Dvt : Inport
  T0 : Inport  Port=2
  Ki : Inport  Port=3
  KiPos : Inport  Port=4
  KiNeg : Inport  Port=5
  WinPos : Inport  Port=6
  WinNeg : Inport  Port=7
  function : TriggerPort  TriggerType=function-call  VariantControl=Variant
  Constant1 : Constant  Value=10  OutDataTypeStr=uint32
  Data Store Read : DataStoreRead  DataStoreName=outputlast1
  Data Store Write : DataStoreWrite  DataStoreName=outputlast1
  Data Type Conversion11 : DataTypeConversion
  Divide2 : Product  Inputs=*/  OutDataTypeStr=fixdt(1,32,2^-16,0)  RndMeth=Round  SaturateOnIntegerOverflow=on
  Product1 : Product  Inputs=*/  OutDataTypeStr=fixdt(1,32,2^-13,0)  RndMeth=Round  SaturateOnIntegerOverflow=on
  Product3 : Product  OutDataTypeStr=fixdt(1,16,2^-7,0)  RndMeth=Round  SaturateOnIntegerOverflow=on
  Relational Operator : RelationalOperator  Operator=>  OutDataTypeStr=boolean  RndMeth=Nearest  InputSameDT=on
  Relational Operator1 : RelationalOperator  Operator=<  OutDataTypeStr=boolean  RndMeth=Nearest  InputSameDT=on
  Sum : Sum  RndMeth=Round  SaturateOnIntegerOverflow=on  InputSameDT=on  OutDataTypeStr=Inherit: Same as first input
  Switch : Switch  Criteria=u2 ~= 0  SaturateOnIntegerOverflow=on  InputSameDT=on
  Switch1 : Switch  Criteria=u2 ~= 0  SaturateOnIntegerOverflow=on  InputSameDT=on
  Out : Outport
  wires:
  Product3/1 -> Sum/2
  Divide2/1 -> Product3/2
  Constant1/1 -> Divide2/2
  Product1/1 -> Divide2/1
  Data Type Conversion11/1 -> Out/1
  Sum/1 -> Data Type Conversion11/1, Data Store Write/1
  Dvt/1 -> Relational Operator1/1, Relational Operator/1, Product3/1
  Switch1/1 -> Product1/1
  T0/1 -> Product1/2
  WinNeg/1 -> Relational Operator1/2
  Ki/1 -> Switch/3
  Data Store Read/1 -> Sum/1
  Switch/1 -> Switch1/3
  WinPos/1 -> Relational Operator/2
  Relational Operator1/1 -> Switch/2
  KiNeg/1 -> Switch/1
  Relational Operator/1 -> Switch1/2
  KiPos/1 -> Switch1/1

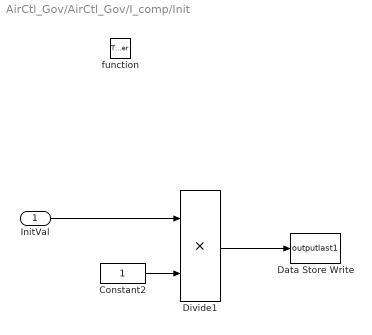
== system AirCtl_Gov/AirCtl_Gov/I_comp/Init ==
  InitVal : Inport
  function : TriggerPort  TriggerType=function-call  VariantControl=Variant
  Constant2 : Constant  OutDataTypeStr=uint32
  Data Store Write : DataStoreWrite  DataStoreName=outputlast1
  Divide1 : Product  Inputs=**  OutDataTypeStr=Inherit: Inherit via back propagation  RndMeth=Round  SaturateOnIntegerOverflow=on
  wires:
  Constant2/1 -> Divide1/2
  Divide1/1 -> Data Store Write/1
  InitVal/1 -> Divide1/1

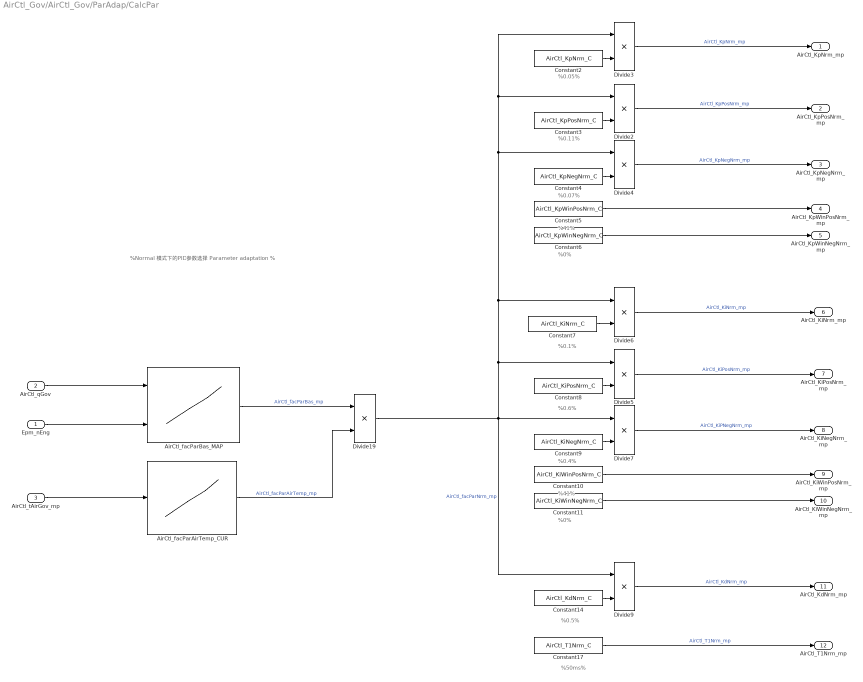
== system AirCtl_Gov/AirCtl_Gov/ParAdap/CalcPar ==
  note: %0.05%
  note: %Normal 模式下的PID参数选择
      | Parameter adaptation %
  note: %0.11%
  note: %0.07%
  note: %41%
  note: %0%
  note: %0.1%
  note: %0.6%
  note: %0.4%
  note: %41%
  note: %0%
  note: %0.5%
  note: %50ms%
  Epm_nEng : Inport
  AirCtl_qGov : Inport  Port=2
  AirCtl_tAirGov_mp : Inport  Port=3
  AirCtl_facParAirTemp_CUR : Lookup_n-D  NumberOfTableDimensions=1  BreakpointsForDimension1=AirCtl_facParAirTemp_CURX  BeginIndexSearchUsingPreviousIndexResult=on  Table=AirCtl_facParAirTemp_CUR  TableDataTypeStr=Inherit: Inherit from 'Table data'  ExtrapMethod=Clip  UseLastTableValue=on  InternalRulePriority=Speed  OutDataTypeStr=Inherit: Inherit from 'Table data'  RndMeth=Simplest  SaturateOnIntegerOverflow=on
  AirCtl_facParBas_MAP : Lookup_n-D  BreakpointsForDimension1=AirCtl_facParBas_MAPY  BreakpointsForDimension2=AirCtl_facParBas_MAPX  BeginIndexSearchUsingPreviousIndexResult=on  Table=AirCtl_facParBas_MAP  TableDataTypeStr=Inherit: Inherit from 'Table data'  ExtrapMethod=Clip  UseLastTableValue=on  InternalRulePriority=Speed  OutDataTypeStr=Inherit: Inherit from 'Table data'  RndMeth=Simplest  SaturateOnIntegerOverflow=on
  Constant10 : Constant  Value=AirCtl_KiWinPosNrm_C  SampleTime=-1
  Constant11 : Constant  Value=AirCtl_KiWinNegNrm_C  SampleTime=-1
  Constant14 : Constant  Value=AirCtl_KdNrm_C
  Constant17 : Constant  Value=AirCtl_T1Nrm_C  SampleTime=-1
  Constant2 : Constant  Value=AirCtl_KpNrm_C
  Constant3 : Constant  Value=AirCtl_KpPosNrm_C
  Constant4 : Constant  Value=AirCtl_KpNegNrm_C
  Constant5 : Constant  Value=AirCtl_KpWinPosNrm_C  SampleTime=-1
  Constant6 : Constant  Value=AirCtl_KpWinNegNrm_C  SampleTime=-1
  Constant7 : Constant  Value=AirCtl_KiNrm_C
  Constant8 : Constant  Value=AirCtl_KiPosNrm_C
  Constant9 : Constant  Value=AirCtl_KiNegNrm_C
  Divide{2..7,9,19} (8 alike) : Product  Inputs=**  OutDataTypeStr=Inherit: Inherit via back propagation  SaturateOnIntegerOverflow=on
  AirCtl_KpNrm_mp : Outport
  AirCtl_KpPosNrm_mp : Outport  Port=2
  AirCtl_KpNegNrm_mp : Outport  Port=3
  AirCtl_KpWinPosNrm_mp : Outport  Port=4
  AirCtl_KpWinNegNrm_mp : Outport  Port=5
  AirCtl_KiNrm_mp : Outport  Port=6
  AirCtl_KiPosNrm_mp : Outport  Port=7
  AirCtl_KiNegNrm_mp : Outport  Port=8
  AirCtl_KiWinPosNrm_mp : Outport  Port=9
  AirCtl_KiWinNegNrm_mp : Outport  Port=10
  AirCtl_KdNrm_mp : Outport  Port=11
  AirCtl_T1Nrm_mp : Outport  Port=12
  wires:
  Constant17/1 -> AirCtl_T1Nrm_mp/1  "AirCtl_T1Nrm_mp"
  Divide9/1 -> AirCtl_KdNrm_mp/1  "AirCtl_KdNrm_mp"
  Constant14/1 -> Divide9/2
  Constant11/1 -> AirCtl_KiWinNegNrm_mp/1
  Constant10/1 -> AirCtl_KiWinPosNrm_mp/1
  Divide7/1 -> AirCtl_KiNegNrm_mp/1  "AirCtl_KiPNegNrm_mp"
  Constant9/1 -> Divide7/2
  Divide5/1 -> AirCtl_KiPosNrm_mp/1  "AirCtl_KiPosNrm_mp"
  Divide6/1 -> AirCtl_KiNrm_mp/1  "AirCtl_KiNrm_mp"
  Constant8/1 -> Divide5/2
  Constant7/1 -> Divide6/2
  Constant6/1 -> AirCtl_KpWinNegNrm_mp/1
  Constant5/1 -> AirCtl_KpWinPosNrm_mp/1
  Divide4/1 -> AirCtl_KpNegNrm_mp/1  "AirCtl_KpNegNrm_mp"
  Constant4/1 -> Divide4/2
  Divide2/1 -> AirCtl_KpPosNrm_mp/1  "AirCtl_KpPosNrm_mp"
  Divide3/1 -> AirCtl_KpNrm_mp/1  "AirCtl_KpNrm_mp"
  Constant3/1 -> Divide2/2
  Constant2/1 -> Divide3/2
  Divide19/1 -> Divide9/1, Divide7/1, Divide6/1, Divide4/1, Divide3/1, Divide2/1, Divide5/1  "AirCtl_facParNrm_mp"
  AirCtl_facParAirTemp_CUR/1 -> Divide19/2  "AirCtl_facParAirTemp_mp"
  AirCtl_facParBas_MAP/1 -> Divide19/1  "AirCtl_facParBas_mp"
  AirCtl_tAirGov_mp/1 -> AirCtl_facParAirTemp_CUR/1
  Epm_nEng/1 -> AirCtl_facParBas_MAP/2
  AirCtl_qGov/1 -> AirCtl_facParBas_MAP/1
